simulink model "untitled"  (R2018b)
settings: Solver=VariableStepAuto  StartTime=0.0  StopTime=5  RelTol=1e-3
libraries: commblkcod2 x2, commrandsrc3 x1, commchan3 x1, commsink2 x1
settings Model: Creator=nhat  LastModifiedBy=nhat

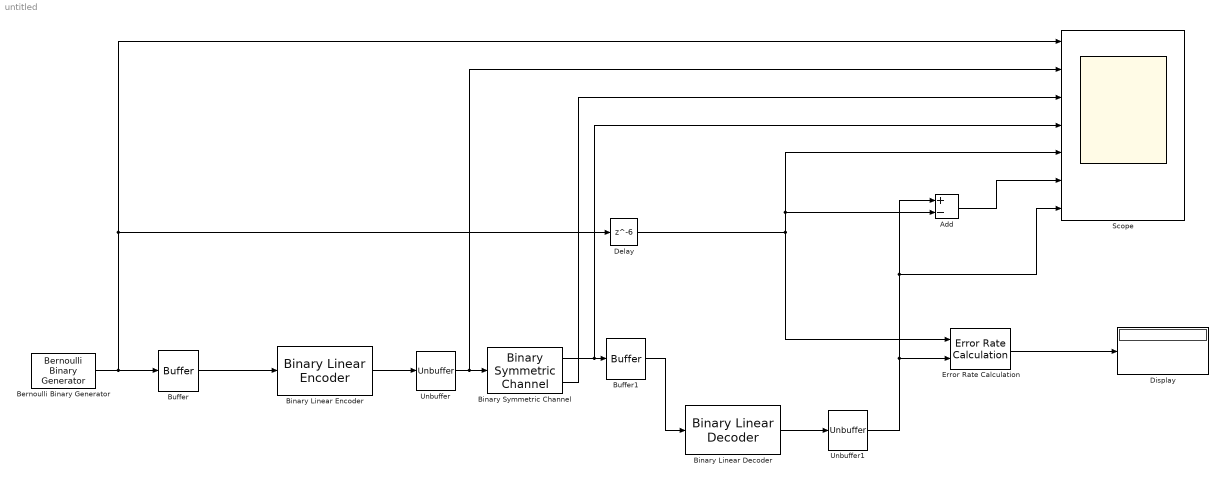
== system untitled ==
  Add : Sum  Inputs=+-
  Bernoulli Binary Generator : commrandsrc3/Bernoulli Binary Generator  ProbabilityOfZero=0.5  SeedSource=Auto  Seed=0  SampleTime=1/1000  SamplesPerFrame=1  OutputDataType=double  SimulateUsing=Interpreted execution
  Binary Linear Decoder : commblkcod2/Binary Linear Decoder  G=[[1 1 0; 0 1 1; 1 0 1] eye(3)]  trt=0
      settings: SourceProductName=Communications System Toolbox  SourceProductBaseCode=CM
  Binary Linear Encoder : commblkcod2/Binary Linear Encoder  G=[[1 1 0; 0 1 1; 1 0 1] eye(3)]
      settings: SourceProductName=Communications System Toolbox  SourceProductBaseCode=CM
  Binary Symmetric Channel : commchan3/Binary Symmetric Channel  ErrorProbability=0.01  ErrorVectorOutputPort=on  OutputDataType=double  OutputDataTypeSL=double  Seed=71  SimulateUsing=Code generation
      settings: SourceProductName=Communications System Toolbox  SourceProductBaseCode=CM
  Buffer : Buffer  N=3  OutputFrames=off
  Buffer1 : Buffer  N=6  OutputFrames=off
  Delay : Delay  DelayLength=6
  Display : Display
  Error Rate Calculation : commsink2/Error Rate Calculation  N=0  st_delay=0  cp_mode=Entire frame  subframe=[]  PMode=Port  WsName=ErrorVec  RsMode2=off  stop=off  numErr=100  maxBits=1e6
  Scope : Scope  NumInputPorts=7
  Unbuffer : Unbuffer
  Unbuffer1 : Unbuffer
  wires:
  Bernoulli Binary Generator/1 -> Scope/1, Delay/1, Buffer/1
  Buffer/1 -> Binary Linear Encoder/1
  Binary Linear Encoder/1 -> Unbuffer/1
  Unbuffer/1 -> Scope/2, Binary Symmetric Channel/1
  Binary Symmetric Channel/1 -> Scope/4, Buffer1/1
  Buffer1/1 -> Binary Linear Decoder/1
  Binary Linear Decoder/1 -> Unbuffer1/1
  Unbuffer1/1 -> Add/1, Scope/7, Error Rate Calculation/2
  Error Rate Calculation/1 -> Display/1
  Delay/1 -> Scope/5, Add/2, Error Rate Calculation/1
  Binary Symmetric Channel/2 -> Scope/3
  Add/1 -> Scope/6
